simulink library "qrd_matrix_library"  (Simulink 8.7)
settings: Solver=ode45  StartTime=0.0  StopTime=10.0  RelTol=1e-3
values from neighbouring files (symbols this model uses):
  vectorization = 2    [qrd_test.m]
undefined symbols (not defined in the file or in its folder): AdvDSPBChannelOutDisplay, AdvDSPBDMemDisplay, Back_Substitution_instances, column_count, column_count_1, column_count_2, dpoly, dspba_ChannelInVis, dspba_ChannelOutVis, dspba_internal_get_channel_ports, evalAionMaskParam, latency, primtype, QRD_vectorization, recipsqrt, row, row_count, row_count_1, row_count_2, UseDontCare, value, x
libraries: DSPBAPrim x683, DSPBAControl x37, qrd_matrix_library x33, DSPBAVectorUtil x6, DSPBAVectorPrim x3
(part 4 of 8)

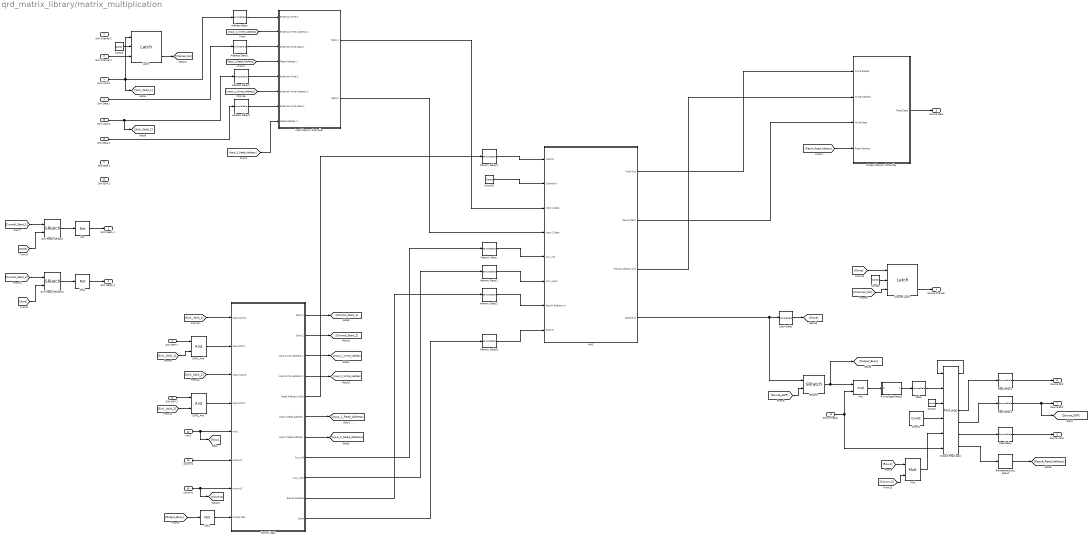
== system qrd_matrix_library/matrix_multiplication ==
  Sink Valid 1 : Inport
  Sink Channel 1 : Inport  Port=2
  Sink Data 1 : Inport  Port=3
  Sink SOP 1 : Inport  Port=4
  Sink EOP 1 : Inport  Port=5
  Sink Valid 2 : Inport  Port=6
  Sink Channel 2 : Inport  Port=7
  Sink Data 2 : Inport  Port=8
  Sink SOP 2 : Inport  Port=9
  Sink EOP 2 : Inport  Port=10
  Source Ready : Inport  Port=11
  row1 : Inport  Port=12
  column1 : Inport  Port=13
  column2 : Inport  Port=14
  Address Delay{,1..3} (4 alike) : DSPBAPrim/SampleDelay  primtype=sampdelay  nInputs=1  nOutputs=1  omode=Inherit via internal rule  otype=sfix(16)  scale=2^-15  rndmethod=Unbiased  factor=1  satmethod=Symmetric  shift_vec=[0 1 2 -1]  value=1  inPortNames=[' '; ' ';]  outPortNames=[' ']  dspbaimage=dspba_prim.jpg  text=dpoly(1, eye(1,value+1), 'z')  style=Optimised  visibilities=8 + 1024 + 2^17 + 2^18  flexible=off  slackgroup=0  augmented=0  version=20090407  advOptions=[]
  And : DSPBAPrim/And  primtype=and  nInputs=2  nOutputs=1  omode=Inherit via internal rule  otype=sfix(16)  scale=2^-15  rndmethod=Unbiased  factor=1  satmethod=Symmetric  shift_vec=[0 1 2 -1]  value=0  inPortNames=[' '; ' '; ' '; ' '; ' '; ' '; ' '; ' '; ' '; ' '; ' '; ' '; ' '; ' '; ' '; ' '; ]  outPortNames=[' ']  dspbaimage=dspba_prim.jpg  text=fprintf('&');  style=Optimised  visibilities=8+2  version=20090407
  Channel Latch : qrd_matrix_library/Latch
  Const1 : DSPBAPrim/Const  primtype=const  nInputs=0  nOutputs=1  omode=Inherit via internal rule  otype=uint(nextpow2(row*row))  scale=1  rndmethod=Unbiased  factor=1  satmethod=Symmetric  shift_vec=[0 1 2 -1]  value=1  inPortNames=['+'; '+';]  outPortNames=[' ']  dspbaimage=dspba_prim.jpg  text=fprintf('%s', num2str(value));  style=Optimised  visibilities=8 + 1024  floatPrecision=float32_m23  version=20120820
  Const2 : DSPBAPrim/Const  primtype=const  nInputs=0  nOutputs=1  omode=Specify via dialog  otype=uint(nextpow2(row_count_1*column_count_2))  scale=1  rndmethod=Unbiased  factor=1  satmethod=Symmetric  shift_vec=[0 1 2 -1]  value=0  inPortNames=['+'; '+';]  outPortNames=[' ']  dspbaimage=dspba_prim.jpg  text=fprintf('%s', num2str(value));  style=Optimised  visibilities=8 + 1024  floatPrecision=float32_m23  version=20120820
  Const26 : DSPBAPrim/Const  primtype=const  nInputs=0  nOutputs=1  omode=Specify via dialog  otype=uint(8)  scale=1  rndmethod=Unbiased  factor=1  satmethod=Symmetric  shift_vec=[0 1 2 -1]  value=0  inPortNames=['+'; '+';]  outPortNames=[' ']  dspbaimage=dspba_prim.jpg  text=fprintf('%s', num2str(value));  style=Optimised  visibilities=8 + 1024  floatPrecision=float32_m23  version=20120820
  Const6 : DSPBAPrim/Const  primtype=const  nInputs=0  nOutputs=1  omode=Specify via dialog  otype=uint(8)  scale=1  rndmethod=Unbiased  factor=1  satmethod=Symmetric  shift_vec=[0 1 2 -1]  value=0  inPortNames=['+'; '+';]  outPortNames=[' ']  dspbaimage=dspba_prim.jpg  text=fprintf('%s', num2str(value));  style=Optimised  visibilities=8 + 1024  floatPrecision=float32_m23  version=20120820
  Const8 : DSPBAPrim/Const  primtype=const  nInputs=0  nOutputs=1  omode=Specify via dialog  otype=uint(8)  scale=1  rndmethod=Unbiased  factor=1  satmethod=Symmetric  shift_vec=[0 1 2 -1]  value=0  inPortNames=['+'; '+';]  outPortNames=[' ']  dspbaimage=dspba_prim.jpg  text=fprintf('%s', num2str(value));  style=Optimised  visibilities=8 + 1024  floatPrecision=float32_m23  version=20120820
  Control Logic : Subsystem  BlockChoice=Row Major Control Logic
      settings: AttributesFormatString=%<BlockChoice>  TemplateBlock=qrd_matrix_library/Control Logic  MemberBlocks=Column Major Control Logic,Row Major Control Logic
  Delay : DSPBAPrim/SampleDelay  primtype=sampdelay  nInputs=1  nOutputs=1  omode=Inherit via internal rule  otype=sfix(16)  scale=2^-15  rndmethod=Unbiased  factor=1  satmethod=Symmetric  shift_vec=[0 1 2 -1]  value=1  inPortNames=[' '; ' ';]  outPortNames=[' ']  dspbaimage=dspba_prim.jpg  text=dpoly(1, eye(1,value+1), 'z')  style=Optimised  visibilities=8 + 1024 + 2^17 + 2^18  flexible=off  slackgroup=0  augmented=0  version=20090407  advOptions=[]
  Input Memory Controller : Subsystem
  Latch : qrd_matrix_library/Latch
  Latch Delay : DSPBAPrim/SampleDelay  primtype=sampdelay  nInputs=1  nOutputs=1  omode=Inherit via internal rule  otype=sfix(16)  scale=2^-15  rndmethod=Unbiased  factor=1  satmethod=Symmetric  shift_vec=[0 1 2 -1]  value=1  inPortNames=[' '; ' ';]  outPortNames=[' ']  dspbaimage=dspba_prim.jpg  text=dpoly(1, eye(1,value+1), 'z')  style=Optimised  visibilities=8 + 1024 + 2^17 + 2^18  flexible=off  slackgroup=0  augmented=0  version=20090407  advOptions=[]
  MAC : Subsystem
  Memory Delay{,1..2,4,6} (5 alike) : DSPBAPrim/SampleDelay  primtype=sampdelay  nInputs=1  nOutputs=1  omode=Inherit via internal rule  otype=sfix(16)  scale=2^-15  rndmethod=Unbiased  factor=1  satmethod=Symmetric  shift_vec=[0 1 2 -1]  value=2  inPortNames=[' '; ' ';]  outPortNames=[' ']  dspbaimage=dspba_prim.jpg  text=dpoly(1, eye(1,value+1), 'z')  style=Optimised  visibilities=8 + 1024 + 2^17 + 2^18  flexible=off  slackgroup=0  augmented=0  version=20090407  advOptions=[]
  Mult : DSPBAPrim/Mult  primtype=mult  nInputs=2  nOutputs=1  omode=Inherit via internal rule  otype=sfix(16)  scale=2^-15  rndmethod=Unbiased  factor=1  satmethod=Symmetric  shift_vec=[0 1 2 -1]  value=0  inPortNames=[' '; ' ';]  outPortNames=[' ']  dspbaimage=dspba_prim.jpg  text=fprintf('X');  style=Optimised  visibilities=8+2^18+2^19  floatPrecision=float32_m23  floatRounding=correct  advOptions=[]  version=20130115
  Not : DSPBAPrim/Not  primtype=not  nInputs=1  nOutputs=1  omode=Inherit via internal rule  otype=sfix(16)  scale=2^-15  rndmethod=Unbiased  factor=1  satmethod=Symmetric  shift_vec=[0 1 2 -1]  value=0  inPortNames=[' '; ' ';]  outPortNames=[' ']  dspbaimage=dspba_prim.jpg  text=fprintf('~');  style=Optimised  visibilities=8  version=20090407
  Not1 : DSPBAPrim/Not  primtype=not  nInputs=1  nOutputs=1  omode=Inherit via internal rule  otype=sfix(16)  scale=2^-15  rndmethod=Unbiased  factor=1  satmethod=Symmetric  shift_vec=[0 1 2 -1]  value=0  inPortNames=[' '; ' ';]  outPortNames=[' ']  dspbaimage=dspba_prim.jpg  text=fprintf('~');  style=Optimised  visibilities=8  version=20090407
  Not2 : DSPBAPrim/Not  primtype=not  nInputs=1  nOutputs=1  omode=Inherit via internal rule  otype=sfix(16)  scale=2^-15  rndmethod=Unbiased  factor=1  satmethod=Symmetric  shift_vec=[0 1 2 -1]  value=0  inPortNames=[' '; ' ';]  outPortNames=[' ']  dspbaimage=dspba_prim.jpg  text=fprintf('~');  style=Optimised  visibilities=8  version=20090407
  Output Memory Controller : Subsystem
  Output Read Logic : DSPBAPrim/ForLoop  looptest=<
  Read Delay : DSPBAPrim/SampleDelay  primtype=sampdelay  nInputs=1  nOutputs=1  omode=Inherit via internal rule  otype=sfix(16)  scale=2^-15  rndmethod=Unbiased  factor=1  satmethod=Symmetric  shift_vec=[0 1 2 -1]  value=2  inPortNames=[' '; ' ';]  outPortNames=[' ']  dspbaimage=dspba_prim.jpg  text=dpoly(1, eye(1,value+1), 'z')  style=Optimised  visibilities=8 + 1024 + 2^17 + 2^18  flexible=off  slackgroup=0  augmented=0  version=20090407  advOptions=[]
  Read Delay1 : DSPBAPrim/SampleDelay  primtype=sampdelay  nInputs=1  nOutputs=1  omode=Inherit via internal rule  otype=sfix(16)  scale=2^-15  rndmethod=Unbiased  factor=1  satmethod=Symmetric  shift_vec=[0 1 2 -1]  value=2  inPortNames=[' '; ' ';]  outPortNames=[' ']  dspbaimage=dspba_prim.jpg  text=dpoly(1, eye(1,value+1), 'z')  style=Optimised  visibilities=8 + 1024 + 2^17 + 2^18  flexible=off  slackgroup=0  augmented=0  version=20090407  advOptions=[]
  Read Delay2 : DSPBAPrim/SampleDelay  primtype=sampdelay  nInputs=1  nOutputs=1  omode=Inherit via internal rule  otype=sfix(16)  scale=2^-15  rndmethod=Unbiased  factor=1  satmethod=Symmetric  shift_vec=[0 1 2 -1]  value=2  inPortNames=[' '; ' ';]  outPortNames=[' ']  dspbaimage=dspba_prim.jpg  text=dpoly(1, eye(1,value+1), 'z')  style=Optimised  visibilities=8 + 1024 + 2^17 + 2^18  flexible=off  slackgroup=0  augmented=0  version=20090407  advOptions=[]
  ReinterpretCast_Result : DSPBAPrim/ReinterpretCast  primtype=reinterpret  nInputs=1  nOutputs=1  omode=Specify via dialog  otype=uint(nextpow2(row_count_1*column_count_2))  scale=1  rndmethod=Unbiased  factor=1  satmethod=Symmetric  shift_vec=[0 1 2 -1]  value=0  inPortNames=[' '; ' ';]  outPortNames=[' ']  dspbaimage=dspba_prim.jpg  text=fprintf('Reinterp\nCast', value);  style=Optimised  visibilities=8  floatPrecision=float32_m23  version=20120601
  Rising Edge Detect : Subsystem  Opaque=on
      mask help:
      | The EdgeDetect component detects edges,
      | under the assumption that initial state
      | of the signal is 0 i.e. a 1 on the input
      | in the first cycle will be detected as
      | an edge.
      mask Help: helpview(dspba.GetHelp('EdgeDetect'));
      mask Display:
      | color('w');
      | image(imread('dspba_fft.jpg'));
      | port_label('input',1,'d');
      | port_label('output',1,'q');
      | text(0.4,0.5,sprintf('RED'));
  SOP1_And : DSPBAPrim/And  primtype=and  nInputs=2  nOutputs=1  omode=Inherit via internal rule  otype=sfix(16)  scale=2^-15  rndmethod=Unbiased  factor=1  satmethod=Symmetric  shift_vec=[0 1 2 -1]  value=0  inPortNames=[' '; ' '; ' '; ' '; ' '; ' '; ' '; ' '; ' '; ' '; ' '; ' '; ' '; ' '; ' '; ' '; ]  outPortNames=[' ']  dspbaimage=dspba_prim.jpg  text=fprintf('&');  style=Optimised  visibilities=8+2  version=20090407
  SOP2_And : DSPBAPrim/And  primtype=and  nInputs=2  nOutputs=1  omode=Inherit via internal rule  otype=sfix(16)  scale=2^-15  rndmethod=Unbiased  factor=1  satmethod=Symmetric  shift_vec=[0 1 2 -1]  value=0  inPortNames=[' '; ' '; ' '; ' '; ' '; ' '; ' '; ' '; ' '; ' '; ' '; ' '; ' '; ' '; ' '; ' '; ]  outPortNames=[' ']  dspbaimage=dspba_prim.jpg  text=fprintf('&');  style=Optimised  visibilities=8+2  version=20090407
  SRlatch : DSPBAControl/SRlatch
  Sink Ready SRlatch : DSPBAControl/SRlatch
  Sink Ready SRlatch1 : DSPBAControl/SRlatch
  Sink Ready 1 : Outport
  Sink Ready 2 : Outport  Port=2
  Source Valid : Outport  Port=3
  Source Channel : Outport  Port=4
  Source Data : Outport  Port=5
  Source SOP : Outport  Port=6
  Source EOP : Outport  Port=7
  wires:
  Read Delay1/1 -> Source SOP/1
  Read Delay/1 -> Source Valid/1
  Control Logic/8(Acc_Init) -> Memory Delay/1
  Memory Delay2/1 -> MAC/7(Result Address In)
  Output Memory Controller/1(Read Data) -> Source Data/1
  Address Delay/1 -> Input Memory Controller/1(External Write 1)
  Sink Data 1/1 -> Address Delay1/1
  Memory Delay/1 -> MAC/5(Acc_Init)
  MAC/3(Result Address Out) -> Output Memory Controller/2(Write Address)
  Control Logic/10(Result Address) -> Memory Delay2/1
  MAC/2(Result Data) -> Output Memory Controller/3(Write Data)
  Control Logic/5(Read Address Valid) -> Memory Delay4/1
  Control Logic/3(Input Write Address 1) -> [Input_1_Write_Address]
  Address Delay1/1 -> Input Memory Controller/3(External Write Data 1)
  Source Ready/1 -> Output Read Logic/6, And/2
  [Input_1_Write_Address] -> Input Memory Controller/2(External Write Address 1)
  Memory Delay4/1 -> MAC/1(Valid In)
  Read Delay2/1 -> [Source_EOP], Source EOP/1
  Control Logic/9(Acc_Valid) -> Memory Delay1/1
  MAC/1(Valid Out) -> Output Memory Controller/1(Write Enable)
  [Result_Read_Address] -> Output Memory Controller/4(Read Address)
  Rising Edge Detect/1(q) -> Delay/1
  SRlatch/1 -> [Output_Busy], And/1
  Sink SOP 1/1 -> SOP1_And/1
  Const26/1 -> MAC/2(Channel In)
  Control Logic/6(Input 1 Read Address) -> [Input_1_Read_Address]
  [Input_1_Read_Address] -> Input Memory Controller/4(Read Address 1)
  [Input_2_Read_Address] -> Input Memory Controller/8(Read Address 2)
  And/1 -> Rising Edge Detect/1(d)
  Memory Delay1/1 -> MAC/6(Acc_Valid)
  Input Memory Controller/2(Data 2) -> MAC/4(Input 2 Data)
  Input Memory Controller/1(Data 1) -> MAC/3(Input 1 Data)
  Sink Valid 1/1 -> [Sink_Valid_1], Address Delay/1, Latch/1
  Delay/1 -> Output Read Logic/2
  MAC/4(Done Out) -> Latch Delay/1, SRlatch/1
  Output Read Logic/6 -> Read Delay/1
  Output Read Logic/7 -> ReinterpretCast_Result/1
  Output Read Logic/4 -> Read Delay1/1
  Output Read Logic/5 -> Read Delay2/1
  Mult/1 -> Output Read Logic/5
  Const1/1 -> Output Read Logic/4
  Const2/1 -> Output Read Logic/3
  Output Read Logic/1 -> Output Read Logic/1
  Control Logic/11(Done) -> Memory Delay6/1
  Memory Delay6/1 -> MAC/8(Done In)
  [Source_EOP] -> SRlatch/2
  row1/1 -> [Row1], Control Logic/5(row1)
  column1/1 -> Control Logic/6(column1)
  Not/1 -> Sink Ready 1/1
  [Done] -> Sink Ready SRlatch/2
  [Row1] -> Mult/1
  Sink Channel 1/1 -> Latch/3
  Const6/1 -> Latch/2
  Latch/3 -> [Channel_Out]
  Sink Ready SRlatch/1 -> Not/1
  [Sink_Valid_1] -> SOP1_And/2
  SOP1_And/1 -> Control Logic/2(Input SOP 1)
  Control Logic/1(Start 1) -> [Control_Start_1]
  [Control_Start_1] -> Sink Ready SRlatch/1
  Not1/1 -> Sink Ready 2/1
  [Done] -> Sink Ready SRlatch1/2
  Sink Ready SRlatch1/1 -> Not1/1
  [Control_Start_2] -> Sink Ready SRlatch1/1
  Address Delay2/1 -> Input Memory Controller/5(External Write 2)
  Sink Valid 2/1 -> [Sink_Valid_2], Address Delay2/1
  Address Delay3/1 -> Input Memory Controller/7(External Write Data 2)
  Sink Data 2/1 -> Address Delay3/1
  [Sink_Valid_2] -> SOP2_And/2
  Sink SOP 2/1 -> SOP2_And/1
  [Sink_Valid_1] -> Control Logic/1(Input Valid 1)
  [Sink_Valid_2] -> Control Logic/3(Input Valid 2)
  SOP2_And/1 -> Control Logic/4(Input SOP 2)
  column2/1 -> [Column2], Control Logic/7(column2)
  [Column2] -> Mult/2
  Control Logic/2(Start 2) -> [Control_Start_2]
  [Input_2_Write_Address] -> Input Memory Controller/6(External Write Address 2)
  Control Logic/4(Input Write Address 2) -> [Input_2_Write_Address]
  Control Logic/7(Input 2 Read Address) -> [Input_2_Read_Address]
  ReinterpretCast_Result/1 -> [Result_Read_Address]
  [Output_Busy] -> Not2/1
  Latch Delay/1 -> [Done]
  Not2/1 -> Control Logic/8(Output Idle)
  [Channel_Out] -> Channel Latch/3
  Const8/1 -> Channel Latch/2
  [Done] -> Channel Latch/1
  Channel Latch/3 -> Source Channel/1

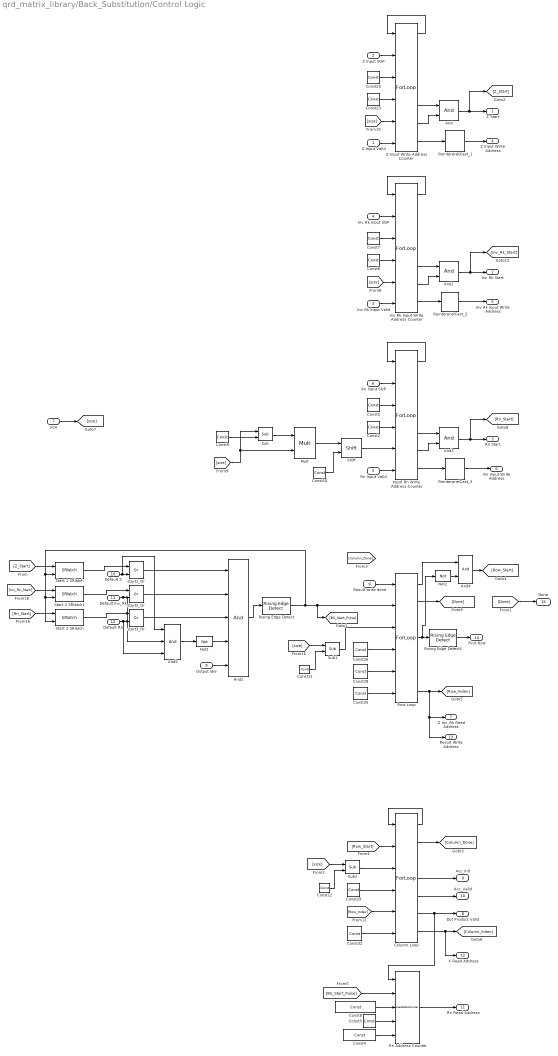
== system qrd_matrix_library/Back_Substitution/Control Logic ==
  Z Input Valid : Inport
  Z Input SOP : Inport  Port=2
  Inv Rk Input Valid : Inport  Port=3
  Inv Rk Input SOP : Inport  Port=4
  Rn Input Valid : Inport  Port=5
  Rn Input SOP : Inport  Port=6
  size : Inport  Port=7
  Output Idle : Inport  Port=8
  Result write done : Inport  Port=9
  Default Z : Inport  Port=10
  Default Inv_Rk : Inport  Port=11
  Default Rn : Inport  Port=12
  And{,1,3..4} (4 alike) : DSPBAPrim/And  primtype=and  nInputs=2  nOutputs=1  omode=Inherit via internal rule  otype=sfix(16)  scale=2^-15  rndmethod=Unbiased  factor=1  satmethod=Symmetric  shift_vec=[0 1 2 -1]  value=0  inPortNames=[' '; ' '; ' '; ' '; ' '; ' '; ' '; ' '; ' '; ' '; ' '; ' '; ' '; ' '; ' '; ' '; ]  outPortNames=[' ']  dspbaimage=dspba_prim.jpg  text=fprintf('&');  style=Optimised  visibilities=8+2  version=20090407
  And2 : DSPBAPrim/And  primtype=and  nInputs=5  nOutputs=1  omode=Inherit via internal rule  otype=sfix(16)  scale=2^-15  rndmethod=Unbiased  factor=1  satmethod=Symmetric  shift_vec=[0 1 2 -1]  value=0  inPortNames=[' '; ' '; ' '; ' '; ' '; ' '; ' '; ' '; ' '; ' '; ' '; ' '; ' '; ' '; ' '; ' '; ]  outPortNames=[' ']  dspbaimage=dspba_prim.jpg  text=fprintf('&');  style=Optimised  visibilities=8+2  version=20090407
  And5 : DSPBAPrim/And  primtype=and  nInputs=3  nOutputs=1  omode=Inherit via internal rule  otype=sfix(16)  scale=2^-15  rndmethod=Unbiased  factor=1  satmethod=Symmetric  shift_vec=[0 1 2 -1]  value=0  inPortNames=[' '; ' '; ' '; ' '; ' '; ' '; ' '; ' '; ' '; ' '; ' '; ' '; ' '; ' '; ' '; ' '; ]  outPortNames=[' ']  dspbaimage=dspba_prim.jpg  text=fprintf('&');  style=Optimised  visibilities=8+2  version=20090407
  Column Loop : DSPBAPrim/ForLoop  looptest=>
  Const10 : DSPBAPrim/Const  primtype=const  nInputs=0  nOutputs=1  omode=Inherit via internal rule  otype=uint(nextpow2(row*row))  scale=1  rndmethod=Unbiased  factor=1  satmethod=Symmetric  shift_vec=[0 1 2 -1]  value=1  inPortNames=['+'; '+';]  outPortNames=[' ']  dspbaimage=dspba_prim.jpg  text=fprintf('%s', num2str(value));  style=Optimised  visibilities=8 + 1024  floatPrecision=float32_m23  version=20120820
  Const{2,6,11..12,23,35} (6 alike) : DSPBAPrim/Const  primtype=const  nInputs=0  nOutputs=1  omode=Inherit via internal rule  otype=uint(8)  scale=1  rndmethod=Unbiased  factor=1  satmethod=Symmetric  shift_vec=[0 1 2 -1]  value=1  inPortNames=['+'; '+';]  outPortNames=[' ']  dspbaimage=dspba_prim.jpg  text=fprintf('%s', num2str(value));  style=Optimised  visibilities=8 + 1024  floatPrecision=float32_m23  version=20120820
  Const{5,7,25,28} (4 alike) : DSPBAPrim/Const  primtype=const  nInputs=0  nOutputs=1  omode=Inherit via internal rule  otype=uint(8)  scale=1  rndmethod=Unbiased  factor=1  satmethod=Symmetric  shift_vec=[0 1 2 -1]  value=0  inPortNames=['+'; '+';]  outPortNames=[' ']  dspbaimage=dspba_prim.jpg  text=fprintf('%s', num2str(value));  style=Optimised  visibilities=8 + 1024  floatPrecision=float32_m23  version=20120820
  Const26 : DSPBAPrim/Const  primtype=const  nInputs=0  nOutputs=1  omode=Inherit via internal rule  otype=uint(8)  scale=1  rndmethod=Unbiased  factor=1  satmethod=Symmetric  shift_vec=[0 1 2 -1]  value=-1  inPortNames=['+'; '+';]  outPortNames=[' ']  dspbaimage=dspba_prim.jpg  text=fprintf('%s', num2str(value));  style=Optimised  visibilities=8 + 1024  floatPrecision=float32_m23  version=20120820
  Const29 : DSPBAPrim/Const  primtype=const  nInputs=0  nOutputs=1  omode=Inherit via internal rule  otype=uint(8)  scale=1  rndmethod=Unbiased  factor=1  satmethod=Symmetric  shift_vec=[0 1 2 -1]  value=-1  inPortNames=['+'; '+';]  outPortNames=[' ']  dspbaimage=dspba_prim.jpg  text=fprintf('%s', num2str(value));  style=Optimised  visibilities=8 + 1024  floatPrecision=float32_m23  version=20120820
  Const3 : DSPBAPrim/Const  primtype=const  nInputs=0  nOutputs=1  omode=Inherit via internal rule  otype=uint(8)  scale=1  rndmethod=Unbiased  factor=1  satmethod=Symmetric  shift_vec=[0 1 2 -1]  value=-1  inPortNames=['+'; '+';]  outPortNames=[' ']  dspbaimage=dspba_prim.jpg  text=fprintf('%s', num2str(value));  style=Optimised  visibilities=8 + 1024  floatPrecision=float32_m23  version=20120820
  Const32 : DSPBAPrim/Const  primtype=const  nInputs=0  nOutputs=1  omode=boolean  otype=uint(8)  scale=1  rndmethod=Unbiased  factor=1  satmethod=Symmetric  shift_vec=[0 1 2 -1]  value=1  inPortNames=['+'; '+';]  outPortNames=[' ']  dspbaimage=dspba_prim.jpg  text=fprintf('%s', num2str(value));  style=Optimised  visibilities=8 + 1024  floatPrecision=float32_m23  version=20120820
  Const4 : DSPBAPrim/Const  primtype=const  nInputs=0  nOutputs=1  omode=Inherit via internal rule  otype=uint(8)  scale=1  rndmethod=Unbiased  factor=1  satmethod=Symmetric  shift_vec=[0 1 2 -1]  value=(size-1)*size/2  inPortNames=['+'; '+';]  outPortNames=[' ']  dspbaimage=dspba_prim.jpg  text=fprintf('%s', num2str(value));  style=Optimised  visibilities=8 + 1024  floatPrecision=float32_m23  version=20120820
  Const8 : DSPBAPrim/Const  primtype=const  nInputs=0  nOutputs=1  omode=Inherit via internal rule  otype=uint(8)  scale=1  rndmethod=Unbiased  factor=1  satmethod=Symmetric  shift_vec=[0 1 2 -1]  value=((size-1)*size/2)-1  inPortNames=['+'; '+';]  outPortNames=[' ']  dspbaimage=dspba_prim.jpg  text=fprintf('%s', num2str(value));  style=Optimised  visibilities=8 + 1024  floatPrecision=float32_m23  version=20120820
  Const9 : DSPBAPrim/Const  primtype=const  nInputs=0  nOutputs=1  omode=Inherit via internal rule  otype=uint(nextpow2(row*row))  scale=1  rndmethod=Unbiased  factor=1  satmethod=Symmetric  shift_vec=[0 1 2 -1]  value=1  inPortNames=['+'; '+';]  outPortNames=[' ']  dspbaimage=dspba_prim.jpg  text=fprintf('%s', num2str(value));  style=Optimised  visibilities=8 + 1024  floatPrecision=float32_m23  version=20120820
  Input Rn Write Address Counter : DSPBAPrim/ForLoop  looptest=<
  Inv Rk Input Write Address Counter : DSPBAPrim/ForLoop  looptest=<
  Mult : DSPBAPrim/Mult  primtype=mult  nInputs=2  nOutputs=1  omode=Inherit via internal rule  otype=sfix(16)  scale=2^-15  rndmethod=Unbiased  factor=1  satmethod=Symmetric  shift_vec=[0 1 2 -1]  value=0  inPortNames=[' '; ' ';]  outPortNames=[' ']  dspbaimage=dspba_prim.jpg  text=fprintf('X');  style=Optimised  visibilities=8+2^18+2^19  floatPrecision=float32_m23  floatRounding=correct  advOptions=[]  version=20130115
  Not1 : DSPBAPrim/Not  primtype=not  nInputs=1  nOutputs=1  omode=Inherit via internal rule  otype=sfix(16)  scale=2^-15  rndmethod=Unbiased  factor=1  satmethod=Symmetric  shift_vec=[0 1 2 -1]  value=0  inPortNames=[' '; ' ';]  outPortNames=[' ']  dspbaimage=dspba_prim.jpg  text=fprintf('~');  style=Optimised  visibilities=8  version=20090407
  Not2 : DSPBAPrim/Not  primtype=not  nInputs=1  nOutputs=1  omode=Inherit via internal rule  otype=sfix(16)  scale=2^-15  rndmethod=Unbiased  factor=1  satmethod=Symmetric  shift_vec=[0 1 2 -1]  value=0  inPortNames=[' '; ' ';]  outPortNames=[' ']  dspbaimage=dspba_prim.jpg  text=fprintf('~');  style=Optimised  visibilities=8  version=20090407
  ReinterpretCast_1 : DSPBAPrim/ReinterpretCast  primtype=reinterpret  nInputs=1  nOutputs=1  omode=Specify via dialog  otype=uint(nextpow2(size))  scale=1  rndmethod=Unbiased  factor=1  satmethod=Symmetric  shift_vec=[0 1 2 -1]  value=0  inPortNames=[' '; ' ';]  outPortNames=[' ']  dspbaimage=dspba_prim.jpg  text=fprintf('Reinterp\nCast', value);  style=Optimised  visibilities=8  floatPrecision=float32_m23  version=20120601
  ReinterpretCast_2 : DSPBAPrim/ReinterpretCast  primtype=reinterpret  nInputs=1  nOutputs=1  omode=Specify via dialog  otype=uint(nextpow2(size))  scale=1  rndmethod=Unbiased  factor=1  satmethod=Symmetric  shift_vec=[0 1 2 -1]  value=0  inPortNames=[' '; ' ';]  outPortNames=[' ']  dspbaimage=dspba_prim.jpg  text=fprintf('Reinterp\nCast', value);  style=Optimised  visibilities=8  floatPrecision=float32_m23  version=20120601
  ReinterpretCast_3 : DSPBAPrim/ReinterpretCast  primtype=reinterpret  nInputs=1  nOutputs=1  omode=Specify via dialog  otype=uint(nextpow2(((size-1)*size/2)))  scale=1  rndmethod=Unbiased  factor=1  satmethod=Symmetric  shift_vec=[0 1 2 -1]  value=0  inPortNames=[' '; ' ';]  outPortNames=[' ']  dspbaimage=dspba_prim.jpg  text=fprintf('Reinterp\nCast', value);  style=Optimised  visibilities=8  floatPrecision=float32_m23  version=20120601
  Rising Edge Detect : qrd_matrix_library/matrix_multiplication/Rising Edge Detect
  Rising Edge Detect1 : qrd_matrix_library/matrix_multiplication/Rising Edge Detect
  Rn Address Counter : DSPBAPrim/LoadableCounter  primtype=loadablecounter  nInputs=5  nOutputs=1  omode=Inherit via internal rule  otype=ufix(16)  scale=2^-0  rndmethod=Unbiased  factor=1  satmethod=Symmetric  shift_vec=[0 1 2 -1]  value=[((size-1)*size/2)-1 ((size-1)*size/2) -1]  inPortNames=['en';'ld';'i ';'s ';'m ']  outPortNames=[' ']  dspbaimage=dspba_prim.jpg  text=fprintf('loadable\ncounter\n[%d %d %d]', value(1), value(2), value(3));  style=Optimised  visibilities=8 + 1024  version=20090407
  Row Loop : DSPBAPrim/ForLoop  looptest=>=
  Shift : DSPBAPrim/Shift  primtype=shift  nInputs=2  nOutputs=1  omode=Inherit via internal rule  otype=uint(nextpow2(((size-1)*size/2)))  scale=1  rndmethod=Unbiased  factor=1  satmethod=Symmetric  shift_vec=[0 1 2 -1]  value=0  inPortNames=['a'; 'b';]  outPortNames=[' ']  dspbaimage=dspba_prim.jpg  text=fprintf('a >> b');  style=Optimised  visibilities=8  version=20090407
  Start 1 SRlatch : DSPBAControl/SRlatch
  Start 2 SRlatch1 : DSPBAControl/SRlatch
  Start 3 SRlatch : DSPBAControl/SRlatch
  Sub : DSPBAPrim/Sub  primtype=sub  nInputs=2  nOutputs=1  omode=Specify via dialog  otype=uint(nextpow2(size))  scale=1  rndmethod=Unbiased  factor=1  satmethod=Symmetric  shift_vec=[0 1 2 -1]  value=0  inPortNames=['+'; '-';]  outPortNames=[' ']  dspbaimage=dspba_prim.jpg  text=fprintf('-');  style=Optimised  visibilities=8+2^17+2^18  floatRounding=correct  advOptions=[]  version=20130115
  Sub1 : DSPBAPrim/Sub  primtype=sub  nInputs=2  nOutputs=1  omode=Inherit via internal rule with word growth  otype=sfix(16)  scale=2^-15  rndmethod=Unbiased  factor=1  satmethod=Symmetric  shift_vec=[0 1 2 -1]  value=0  inPortNames=['+'; '-';]  outPortNames=[' ']  dspbaimage=dspba_prim.jpg  text=fprintf('-');  style=Optimised  visibilities=8+2^17+2^18  floatRounding=correct  advOptions=[]  version=20130115
  Sub2 : DSPBAPrim/Sub  primtype=sub  nInputs=2  nOutputs=1  omode=Inherit via internal rule with word growth  otype=sfix(16)  scale=2^-15  rndmethod=Unbiased  factor=1  satmethod=Symmetric  shift_vec=[0 1 2 -1]  value=0  inPortNames=['+'; '-';]  outPortNames=[' ']  dspbaimage=dspba_prim.jpg  text=fprintf('-');  style=Optimised  visibilities=8+2^17+2^18  floatRounding=correct  advOptions=[]  version=20130115
  Z Input Write Address Counter : DSPBAPrim/ForLoop  looptest=<
  start1_Or : DSPBAPrim/Or  primtype=or  nInputs=2  nOutputs=1  omode=Inherit via internal rule  otype=sfix(16)  scale=2^-15  rndmethod=Unbiased  factor=1  satmethod=Symmetric  shift_vec=[0 1 2 -1]  value=0  inPortNames=[' '; ' '; ' '; ' '; ' '; ' '; ' '; ' '; ' '; ' '; ' '; ' '; ' '; ' '; ' '; ' '; ]  outPortNames=[' ']  dspbaimage=dspba_prim.jpg  text=fprintf('|');  style=Optimised  visibilities=8+2  version=20090407
  start2_Or : DSPBAPrim/Or  primtype=or  nInputs=2  nOutputs=1  omode=Inherit via internal rule  otype=sfix(16)  scale=2^-15  rndmethod=Unbiased  factor=1  satmethod=Symmetric  shift_vec=[0 1 2 -1]  value=0  inPortNames=[' '; ' '; ' '; ' '; ' '; ' '; ' '; ' '; ' '; ' '; ' '; ' '; ' '; ' '; ' '; ' '; ]  outPortNames=[' ']  dspbaimage=dspba_prim.jpg  text=fprintf('|');  style=Optimised  visibilities=8+2  version=20090407
  start3_Or : DSPBAPrim/Or  primtype=or  nInputs=2  nOutputs=1  omode=Inherit via internal rule  otype=sfix(16)  scale=2^-15  rndmethod=Unbiased  factor=1  satmethod=Symmetric  shift_vec=[0 1 2 -1]  value=0  inPortNames=[' '; ' '; ' '; ' '; ' '; ' '; ' '; ' '; ' '; ' '; ' '; ' '; ' '; ' '; ' '; ' '; ]  outPortNames=[' ']  dspbaimage=dspba_prim.jpg  text=fprintf('|');  style=Optimised  visibilities=8+2  version=20090407
  Z Start : Outport
  Inv Rk Start : Outport  Port=2
  Rn Start : Outport  Port=3
  Z Input Write Address : Outport  Port=4
  Inv Rk Input Write Address : Outport  Port=5
  Rn Input Write Address : Outport  Port=6
  Z Inv_Rk Read Address : Outport  Port=7
  Dot Product Valid : Outport  Port=8
  Acc_Init : Outport  Port=9
  Acc_Valid : Outport  Port=10
  Rn Read Address : Outport  Port=11
  X Read Address : Outport  Port=12
  Result Write Address : Outport  Port=13
  First Row : Outport  Port=14
  Done : Outport  Port=15
  wires:
  Z Input SOP/1 -> Z Input Write Address Counter/2
  Z Input Write Address Counter/6 -> And/2
  Z Input Write Address Counter/5 -> And/1
  Z Input Write Address Counter/1 -> Z Input Write Address Counter/1
  Z Input Valid/1 -> Z Input Write Address Counter/6
  size/1 -> [size]
  Row Loop/2 -> [Done]
  Column Loop/7 -> X Read Address/1, [Column_Index]
  Row Loop/1 -> And4/1
  [Row_Start] -> Column Loop/2
  Result write done/1 -> Row Loop/1
  Column Loop/2 -> [Column_Done]
  Column Loop/1 -> Column Loop/1
  Const35/1 -> Row Loop/6
  Const32/1 -> Column Loop/6
  Row Loop/7 -> Result Write Address/1, Z Inv_Rk Read Address/1, [Row_Index]
  Rising Edge Detect/1 -> [BS_Start_Pulse], Row Loop/2, Start 1 SRlatch/2, Start 3 SRlatch/2, Start 2 SRlatch1/2
  Const29/1 -> Column Loop/4
  [Row_Index] -> Column Loop/5
  Const26/1 -> Row Loop/4
  Const28/1 -> Row Loop/5
  Z Input Write Address Counter/7 -> ReinterpretCast_1/1
  Const25/1 -> Z Input Write Address Counter/3
  Const23/1 -> Z Input Write Address Counter/4
  Inv Rk Input SOP/1 -> Inv Rk Input Write Address Counter/2
  Inv Rk Input Write Address Counter/6 -> And1/2
  Inv Rk Input Write Address Counter/5 -> And1/1
  Inv Rk Input Write Address Counter/1 -> Inv Rk Input Write Address Counter/1
  Inv Rk Input Valid/1 -> Inv Rk Input Write Address Counter/6
  Inv Rk Input Write Address Counter/7 -> ReinterpretCast_2/1
  Const7/1 -> Inv Rk Input Write Address Counter/3
  Const6/1 -> Inv Rk Input Write Address Counter/4
  And/1 -> [Z_Start], Z Start/1
  And1/1 -> [Inv_Rk_Start], Inv Rk Start/1
  [Z_Start] -> Start 1 SRlatch/1
  [Inv_Rk_Start] -> Start 2 SRlatch1/1
  And2/1 -> Rising Edge Detect/1
  Sub2/1 -> Column Loop/3
  ReinterpretCast_1/1 -> Z Input Write Address/1
  ReinterpretCast_2/1 -> Inv Rk Input Write Address/1
  Start 3 SRlatch/1 -> start3_Or/1
  Start 1 SRlatch/1 -> start1_Or/1
  Start 2 SRlatch1/1 -> start2_Or/1
  [size] -> Z Input Write Address Counter/5
  [size] -> Inv Rk Input Write Address Counter/5
  Rn Input SOP/1 -> Input Rn Write Address Counter/2
  Input Rn Write Address Counter/6 -> And3/2
  Input Rn Write Address Counter/5 -> And3/1
  Input Rn Write Address Counter/1 -> Input Rn Write Address Counter/1
  Rn Input Valid/1 -> Input Rn Write Address Counter/6
  Input Rn Write Address Counter/7 -> ReinterpretCast_3/1
  Const5/1 -> Input Rn Write Address Counter/3
  Const2/1 -> Input Rn Write Address Counter/4
  And3/1 -> Rn Start/1, [Rn_Start]
  ReinterpretCast_3/1 -> Rn Input Write Address/1
  Shift/1 -> Input Rn Write Address Counter/5
  Mult/1 -> Shift/1
  [size] -> Sub/1, Mult/2
  Sub/1 -> Mult/1
  Const9/1 -> Sub/2
  Const10/1 -> Shift/2
  Not1/1 -> And2/4
  [Rn_Start] -> Start 3 SRlatch/1
  [size] -> Sub1/1
  Sub1/1 -> Row Loop/3
  Const11/1 -> Sub1/2
  [size] -> Sub2/1
  Const12/1 -> Sub2/2
  [Done] -> Done/1
  Column Loop/6 -> Rn Address Counter/1, Dot Product Valid/1
  Const3/1 -> Rn Address Counter/4
  Const4/1 -> Rn Address Counter/5
  Const8/1 -> Rn Address Counter/3
  [BS_Start_Pulse] -> Rn Address Counter/2
  Rn Address Counter/1 -> Rn Read Address/1
  Row Loop/4 -> Not2/1, Rising Edge Detect1/1
  Rising Edge Detect1/1 -> First Row/1
  Not2/1 -> And4/2
  And4/1 -> [Row_Start]
  Column Loop/4 -> Acc_Init/1
  Column Loop/5 -> Acc_Valid/1
  Default Z/1 -> And5/1, start1_Or/2
  start1_Or/1 -> And2/1
  start2_Or/1 -> And2/2
  Default Inv_Rk/1 -> And5/2, start2_Or/2
  Default Rn/1 -> And5/3, start3_Or/2
  start3_Or/1 -> And2/3
  Output Idle/1 -> And2/5
  And5/1 -> Not1/1

== system qrd_matrix_library/Back_Substitution/Data Mux ==
  Valid In : Inport
  Channel In : Inport  Port=2
  Dot_Product_valid_in : Inport  Port=3
  Divide_valid_in : Inport  Port=4
  First_Column_in : Inport  Port=5
  Rn_Data : Inport  Port=6
  X_Data : Inport  Port=7
  Sub_Data : Inport  Port=8
  Inv_Rk_Data : Inport  Port=9
  Acc_Init_In : Inport  Port=10
  Acc_Valid_In : Inport  Port=11
  Z_Data_In : Inport  Port=12
  ChannelIn : DSPBAPrim/ChannelIn  primtype=channelin  nInputs=dspba_internal_get_channel_ports(gcb)  nOutputs=dspba_internal_get_channel_ports(gcb)  omode=Inherit via internal rule  otype=sfix(16)  scale=2^-15  rndmethod=Unbiased  factor=1  satmethod=Symmetric  shift_vec=[0 1 2 -1]  value=10  inPortNames=['v'; 'c'; '0'; '1'; '2'; '3'; '4'; '5'; '6'; '7'; '8'; '9'; 'A'; 'B'; 'D'; 'E'; 'F'; 'G'; 'H'; 'I'; 'J'; 'K'; 'L'; 'M'; 'N'; 'O'; 'P'; 'Q'; 'R'; 'S'; 'T'; 'U'; 'W'; 'X'; 'Y'; 'Z']  outPortNames=['v'; 'c'; '0'; '1'; '2'; '3'; '4'; '5'; '6'; '7'; '8'; '9'; 'A'; 'B'; 'D'; 'E'; 'F'; 'G'; 'H'; 'I'; 'J'; 'K'; 'L'; 'M'; 'N'; 'O'; 'P'; 'Q'; 'R'; 'S'; 'T'; 'U'; 'W'; 'X'; 'Y'; 'Z']  dspbaimage=dspba_prim.jpg  text=fprintf('In');  style=Optimised  dataSignals=10  foldingEnabled=off  channels=1  sampleRate=200  packetBeginPresent=off  packetBeginEnabled=off  visibilities=dspba_ChannelInVis(gcb)  latencyCorrection=0  version=20141013
  ChannelOut : DSPBAPrim/ChannelOut  primtype=channelout  nInputs=dspba_internal_get_channel_ports(gcb)  nOutputs=dspba_internal_get_channel_ports(gcb)  omode=Inherit via internal rule  otype=sfix(16)  scale=2^-15  rndmethod=Unbiased  factor=1  satmethod=Symmetric  shift_vec=[0 1 2 -1]  value=6  inPortNames=['v'; 'c'; '0'; '1'; '2'; '3'; '4'; '5'; '6'; '7'; '8'; '9'; 'A'; 'B'; 'D'; 'E'; 'F'; 'G'; 'H'; 'I'; 'J'; 'K'; 'L'; 'M'; 'N'; 'O'; 'P'; 'Q'; 'R'; 'S'; 'T'; 'U'; 'W'; 'X'; 'Y'; 'Z']  outPortNames=['v'; 'c'; '0'; '1'; '2'; '3'; '4'; '5'; '6'; '7'; '8'; '9'; 'A'; 'B'; 'D'; 'E'; 'F'; 'G'; 'H'; 'I'; 'J'; 'K'; 'L'; 'M'; 'N'; 'O'; 'P'; 'Q'; 'R'; 'S'; 'T'; 'U'; 'W'; 'X'; 'Y'; 'Z']  dspbaimage=dspba_prim.jpg  text=fprintf('Out%s', AdvDSPBChannelOutDisplay(latency));  style=Optimised  dataSignals=6  foldingEnabled=off  channels=1  sampleRate=200  packetBeginPresent=off  packetBeginEnabled=off  visibilities=dspba_ChannelOutVis(gcb)  latency=0  latencyCorrection=0  version=20141013
  Data1 Select : DSPBAPrim/Select  primtype=select  nInputs=str2num(get_param(gcb,'value'))*2+1  nOutputs=1  omode=Inherit via internal rule  otype=sfix(16)  scale=2^-15  rndmethod=Unbiased  factor=1  satmethod=Symmetric  shift_vec=[0 1 2 -1]  value=2  inPortNames=['d'; '0'; 'a'; '1'; 'b'; '2'; 'c'; '3'; 'd'; '4'; 'e'; '5'; 'f'; '6'; 'g'; '7'; 'h'; '8'; 'i'; '9'; 'j']  outPortNames=[' ']  dspbaimage=dspba_prim.jpg  text=fprintf('%s', primtype);  style=Optimised  visibilities=8 + 1024  version=20090407
  Data2 Select : DSPBAPrim/Select  primtype=select  nInputs=str2num(get_param(gcb,'value'))*2+1  nOutputs=1  omode=Inherit via internal rule  otype=sfix(16)  scale=2^-15  rndmethod=Unbiased  factor=1  satmethod=Symmetric  shift_vec=[0 1 2 -1]  value=2  inPortNames=['d'; '0'; 'a'; '1'; 'b'; '2'; 'c'; '3'; 'd'; '4'; 'e'; '5'; 'f'; '6'; 'g'; '7'; 'h'; '8'; 'i'; '9'; 'j']  outPortNames=[' ']  dspbaimage=dspba_prim.jpg  text=fprintf('%s', primtype);  style=Optimised  visibilities=8 + 1024  version=20090407
  SynthesisInfo : DSPBAPrim/SynthesisInfo  primtype=synthinfo  nInputs=0  nOutputs=0  omode=Inherit via internal rule  otype=sfix(16)  scale=2^-15  rndmethod=Truncate  factor=1  satmethod=Symmetric  shift_vec=[0 1 2 -1]  value=99  inPortNames=[' '; ' ';]  outPortNames=[' ']  dspbaimage=dspba_prim_ctrl.jpg  text=fprintf('Style=%s', style);  style=Scheduled  visibilities=2^17+2^18+2^19+2^20  constraintInUse=off  constraintRelation=>  constraintLimit=2  bitAccurate=off  version=20150220
  Valid_Or : DSPBAPrim/Or  primtype=or  nInputs=2  nOutputs=1  omode=Inherit via internal rule  otype=sfix(16)  scale=2^-15  rndmethod=Unbiased  factor=1  satmethod=Symmetric  shift_vec=[0 1 2 -1]  value=0  inPortNames=[' '; ' '; ' '; ' '; ' '; ' '; ' '; ' '; ' '; ' '; ' '; ' '; ' '; ' '; ' '; ' '; ]  outPortNames=[' ']  dspbaimage=dspba_prim.jpg  text=fprintf('|');  style=Optimised  visibilities=8+2  version=20090407
  Valid Out : Outport
  Data Out 1 : Outport  Port=2
  Data Out 2 : Outport  Port=3
  Acc_Init_Out : Outport  Port=4
  Acc_Valid_Out : Outport  Port=5
  Dot_Product_valid_out : Outport  Port=6
  Divide_Valid_Out : Outport  Port=7
  wires:
  First_Column_in/1 -> ChannelIn/5
  Divide_valid_in/1 -> ChannelIn/4
  Dot_Product_valid_in/1 -> ChannelIn/3
  Sub_Data/1 -> ChannelIn/8
  ChannelOut/1 -> Valid Out/1
  ChannelOut/4 -> Data Out 2/1
  Channel In/1 -> ChannelIn/2
  ChannelOut/5 -> Acc_Init_Out/1
  ChannelOut/3 -> Data Out 1/1
  Data1 Select/1 -> ChannelOut/3
  ChannelOut/6 -> Acc_Valid_Out/1
  Z_Data_In/1 -> ChannelIn/10
  Data2 Select/1 -> ChannelOut/4
  Inv_Rk_Data/1 -> ChannelIn/9
  X_Data/1 -> ChannelIn/7
  Rn_Data/1 -> ChannelIn/6
  Valid In/1 -> ChannelIn/1
  ChannelIn/1 -> ChannelOut/1
  ChannelIn/2 -> ChannelOut/2
  ChannelIn/3 -> Data1 Select/2, ChannelOut/7, Data2 Select/2
  ChannelIn/4 -> Data1 Select/4, Valid_Or/2, Data2 Select/4
  ChannelIn/6 -> Data1 Select/3
  ChannelIn/7 -> Data2 Select/3
  ChannelIn/8 -> Data1 Select/5
  ChannelIn/9 -> Data2 Select/1, Data2 Select/5
  ChannelIn/11 -> ChannelOut/5
  ChannelIn/12 -> ChannelOut/6
  ChannelOut/7 -> Dot_Product_valid_out/1
  Acc_Init_In/1 -> ChannelIn/11
  ChannelIn/5 -> Valid_Or/1
  Valid_Or/1 -> ChannelOut/8
  Acc_Valid_In/1 -> ChannelIn/12
  ChannelIn/10 -> Data1 Select/1
  ChannelOut/8 -> Divide_Valid_Out/1

== system qrd_matrix_library/Back_Substitution/Dot Product ==
  Valid_In : Inport
  Channel_In : Inport  Port=2
  Data_In1 : Inport  Port=3
  Data_In2 : Inport  Port=4
  Acc_Init : Inport  Port=5
  Acc_Valid : Inport  Port=6
  Dot_Product_Valid_In : Inport  Port=7
  Mult_Valid_In : Inport  Port=8
  Acc : DSPBAPrim/Acc  primtype=acc  nInputs=2  nOutputs=4  omode=Inherit via internal rule  otype=sfix(16)  scale=2^-15  rndmethod=Unbiased  factor=1  satmethod=Symmetric  shift_vec=[0 1 2 -1]  value=[-26 20 12]  inPortNames=['x';'n']  outPortNames=['r ';'xO';'xU';'aO';]  dspbaimage=dspba_prim_float.jpg  text=fprintf('acc(x)');  style=Optimised  visibilities=1024  version=20090407
  And : DSPBAPrim/And  primtype=and  nInputs=3  nOutputs=1  omode=Inherit via internal rule  otype=sfix(16)  scale=2^-15  rndmethod=Unbiased  factor=1  satmethod=Symmetric  shift_vec=[0 1 2 -1]  value=0  inPortNames=[' '; ' '; ' '; ' '; ' '; ' '; ' '; ' '; ' '; ' '; ' '; ' '; ' '; ' '; ' '; ' '; ]  outPortNames=[' ']  dspbaimage=dspba_prim.jpg  text=fprintf('&');  style=Optimised  visibilities=8+2  version=20090407
  ChannelIn : DSPBAPrim/ChannelIn  primtype=channelin  nInputs=dspba_internal_get_channel_ports(gcb)  nOutputs=dspba_internal_get_channel_ports(gcb)  omode=Inherit via internal rule  otype=sfix(16)  scale=2^-15  rndmethod=Unbiased  factor=1  satmethod=Symmetric  shift_vec=[0 1 2 -1]  value=6  inPortNames=['v'; 'c'; '0'; '1'; '2'; '3'; '4'; '5'; '6'; '7'; '8'; '9'; 'A'; 'B'; 'D'; 'E'; 'F'; 'G'; 'H'; 'I'; 'J'; 'K'; 'L'; 'M'; 'N'; 'O'; 'P'; 'Q'; 'R'; 'S'; 'T'; 'U'; 'W'; 'X'; 'Y'; 'Z']  outPortNames=['v'; 'c'; '0'; '1'; '2'; '3'; '4'; '5'; '6'; '7'; '8'; '9'; 'A'; 'B'; 'D'; 'E'; 'F'; 'G'; 'H'; 'I'; 'J'; 'K'; 'L'; 'M'; 'N'; 'O'; 'P'; 'Q'; 'R'; 'S'; 'T'; 'U'; 'W'; 'X'; 'Y'; 'Z']  dspbaimage=dspba_prim.jpg  text=fprintf('In');  style=Optimised  dataSignals=6  foldingEnabled=off  channels=1  sampleRate=200  packetBeginPresent=off  packetBeginEnabled=off  visibilities=dspba_ChannelInVis(gcb)  latencyCorrection=0  version=20141013
  Complex to Real-Imag : ComplexToRealImag
  Const7 : DSPBAPrim/Const  primtype=const  nInputs=0  nOutputs=1  omode=Specify via dialog  otype=uint(8)  scale=1  rndmethod=Unbiased  factor=1  satmethod=Symmetric  shift_vec=[0 1 2 -1]  value=0  inPortNames=['+'; '+';]  outPortNames=[' ']  dspbaimage=dspba_prim.jpg  text=fprintf('%s', num2str(value));  style=Optimised  visibilities=8 + 1024  floatPrecision=float32_m23  version=20120820
  Demux : Demux  Outputs=2
  Dot Product ChannelOut : DSPBAPrim/ChannelOut  primtype=channelout  nInputs=dspba_internal_get_channel_ports(gcb)  nOutputs=dspba_internal_get_channel_ports(gcb)  omode=Inherit via internal rule  otype=sfix(16)  scale=2^-15  rndmethod=Unbiased  factor=1  satmethod=Symmetric  shift_vec=[0 1 2 -1]  value=1  inPortNames=['v'; 'c'; '0'; '1'; '2'; '3'; '4'; '5'; '6'; '7'; '8'; '9'; 'A'; 'B'; 'D'; 'E'; 'F'; 'G'; 'H'; 'I'; 'J'; 'K'; 'L'; 'M'; 'N'; 'O'; 'P'; 'Q'; 'R'; 'S'; 'T'; 'U'; 'W'; 'X'; 'Y'; 'Z']  outPortNames=['v'; 'c'; '0'; '1'; '2'; '3'; '4'; '5'; '6'; '7'; '8'; '9'; 'A'; 'B'; 'D'; 'E'; 'F'; 'G'; 'H'; 'I'; 'J'; 'K'; 'L'; 'M'; 'N'; 'O'; 'P'; 'Q'; 'R'; 'S'; 'T'; 'U'; 'W'; 'X'; 'Y'; 'Z']  dspbaimage=dspba_prim.jpg  text=fprintf('Out%s', AdvDSPBChannelOutDisplay(latency));  style=Optimised  dataSignals=1  foldingEnabled=off  channels=1  sampleRate=200  packetBeginPresent=off  packetBeginEnabled=off  visibilities=dspba_ChannelOutVis(gcb)  latency=0  latencyCorrection=0  version=20141013
  Mult : DSPBAPrim/Mult  primtype=mult  nInputs=2  nOutputs=1  omode=Inherit via internal rule  otype=sfix(16)  scale=2^-15  rndmethod=Unbiased  factor=1  satmethod=Symmetric  shift_vec=[0 1 2 -1]  value=0  inPortNames=[' '; ' ';]  outPortNames=[' ']  dspbaimage=dspba_prim.jpg  text=fprintf('X');  style=Optimised  visibilities=8+2^18+2^19  floatPrecision=float32_m23  floatRounding=correct  advOptions=[]  version=20130115
  Mult ChannelOut : DSPBAPrim/ChannelOut  primtype=channelout  nInputs=dspba_internal_get_channel_ports(gcb)  nOutputs=dspba_internal_get_channel_ports(gcb)  omode=Inherit via internal rule  otype=sfix(16)  scale=2^-15  rndmethod=Unbiased  factor=1  satmethod=Symmetric  shift_vec=[0 1 2 -1]  value=1  inPortNames=['v'; 'c'; '0'; '1'; '2'; '3'; '4'; '5'; '6'; '7'; '8'; '9'; 'A'; 'B'; 'D'; 'E'; 'F'; 'G'; 'H'; 'I'; 'J'; 'K'; 'L'; 'M'; 'N'; 'O'; 'P'; 'Q'; 'R'; 'S'; 'T'; 'U'; 'W'; 'X'; 'Y'; 'Z']  outPortNames=['v'; 'c'; '0'; '1'; '2'; '3'; '4'; '5'; '6'; '7'; '8'; '9'; 'A'; 'B'; 'D'; 'E'; 'F'; 'G'; 'H'; 'I'; 'J'; 'K'; 'L'; 'M'; 'N'; 'O'; 'P'; 'Q'; 'R'; 'S'; 'T'; 'U'; 'W'; 'X'; 'Y'; 'Z']  dspbaimage=dspba_prim.jpg  text=fprintf('Out%s', AdvDSPBChannelOutDisplay(latency));  style=Optimised  dataSignals=1  foldingEnabled=off  channels=1  sampleRate=200  packetBeginPresent=off  packetBeginEnabled=off  visibilities=dspba_ChannelOutVis(gcb)  latency=0  latencyCorrection=0  version=20141013
  Mux : Mux  Inputs=2
  Real-Imag to Complex : RealImagToComplex
  ReinterpretCast : DSPBAPrim/ReinterpretCast  primtype=reinterpret  nInputs=1  nOutputs=1  omode=single  otype=sfix(16)  scale=2^-15  rndmethod=Unbiased  factor=1  satmethod=Symmetric  shift_vec=[0 1 2 -1]  value=0  inPortNames=[' '; ' ';]  outPortNames=[' ']  dspbaimage=dspba_prim.jpg  text=fprintf('Reinterp\nCast', value);  style=Optimised  visibilities=8  floatPrecision=float32_m23  version=20120601
  ReinterpretCast1 : DSPBAPrim/ReinterpretCast  primtype=reinterpret  nInputs=1  nOutputs=1  omode=single  otype=sfix(16)  scale=2^-15  rndmethod=Unbiased  factor=1  satmethod=Symmetric  shift_vec=[0 1 2 -1]  value=0  inPortNames=[' '; ' ';]  outPortNames=[' ']  dspbaimage=dspba_prim.jpg  text=fprintf('Reinterp\nCast', value);  style=Optimised  visibilities=8  floatPrecision=float32_m23  version=20120601
  SynthesisInfo : DSPBAPrim/SynthesisInfo  primtype=synthinfo  nInputs=0  nOutputs=0  omode=Inherit via internal rule  otype=sfix(16)  scale=2^-15  rndmethod=Truncate  factor=1  satmethod=Symmetric  shift_vec=[0 1 2 -1]  value=99  inPortNames=[' '; ' ';]  outPortNames=[' ']  dspbaimage=dspba_prim_ctrl.jpg  text=fprintf('Style=%s', style);  style=Scheduled  visibilities=2^17+2^18+2^19+2^20  constraintInUse=off  constraintRelation=>  constraintLimit=2  bitAccurate=off  version=20150220
  latch_0L : DSPBAControl/latch_0L
  Dot Product Valid_Out : Outport
  Dot Product Data_Out : Outport  Port=2
  Mult Valid_out : Outport  Port=3
  Mult Data_out : Outport  Port=4
  wires:
  latch_0L/1 -> Dot Product ChannelOut/3
  ReinterpretCast/1 -> latch_0L/2
  ChannelIn/8 -> Mult ChannelOut/1
  Mult ChannelOut/3 -> Mult Data_out/1
  Mult ChannelOut/1 -> Mult Valid_out/1
  ChannelIn/1 -> And/1
  Const7/1 -> Mult ChannelOut/2
  ChannelIn/2 -> Dot Product ChannelOut/2
  Data_In2/1 -> ChannelIn/4
  Dot Product ChannelOut/3 -> Dot Product Data_Out/1
  Dot Product ChannelOut/1 -> Dot Product Valid_Out/1
  ChannelIn/3 -> Mult/1
  Demux/1 -> Real-Imag to Complex/1
  Acc_Valid/1 -> ChannelIn/6
  Complex to Real-Imag/1 -> Mux/1
  Acc_Init/1 -> ChannelIn/5
  Real-Imag to Complex/1 -> ReinterpretCast/1
  Mult/1 -> Complex to Real-Imag/1, ReinterpretCast1/1
  Complex to Real-Imag/2 -> Mux/2
  Channel_In/1 -> ChannelIn/2
  ChannelIn/4 -> Mult/2
  Acc/1 -> Demux/1
  Mux/1 -> Acc/1
  Demux/2 -> Real-Imag to Complex/2
  ChannelIn/5 -> Acc/2
  Valid_In/1 -> ChannelIn/1
  Data_In1/1 -> ChannelIn/3
  ChannelIn/6 -> And/2, latch_0L/1
  And/1 -> Dot Product ChannelOut/1
  Mult_Valid_In/1 -> ChannelIn/8
  ReinterpretCast1/1 -> Mult ChannelOut/3
  Dot_Product_Valid_In/1 -> ChannelIn/7
  ChannelIn/7 -> And/3

== system qrd_matrix_library/Back_Substitution/Input Memory Controller ==
  Z External Write : Inport
  Z External Write Address : Inport  Port=2
  Z External Write Data : Inport  Port=3
  Z Read Address : Inport  Port=4
  Inv Rk External Write : Inport  Port=5
  Inv Rk External Write Address : Inport  Port=6
  Inv Rk External Write Data : Inport  Port=7
  Inv Rk Read Address : Inport  Port=8
  Rn External Write : Inport  Port=9
  Rn External Write Address : Inport  Port=10
  Rn External Write Data : Inport  Port=11
  Rn Read Address : Inport  Port=12
  Inv Rk Input RAM : DSPBAPrim/DualMem  primtype=dualmem  nInputs=4  nOutputs=2  omode=Inherit via internal rule  otype=sfix(16)  scale=2^-15  rndmethod=Unbiased  factor=1  satmethod=Symmetric  shift_vec=[0 1 2 -1]  value=(zeros(size,1))  inPortNames=['d1'; 'a1'; 'w1'; 'a2']  outPortNames=['q1'; 'q2']  dspbaimage=dspba_prim.jpg  text=fprintf('dmem%s',AdvDSPBDMemDisplay(UseDontCare));  style=Optimised  visibilities=8 + 1024 + 2^17 + 2^18  UseDontCare=on  TwinWritePorts=off  version=20141001
  Rn Input RAM : DSPBAPrim/DualMem  primtype=dualmem  nInputs=4  nOutputs=2  omode=Inherit via internal rule  otype=sfix(16)  scale=2^-15  rndmethod=Unbiased  factor=1  satmethod=Symmetric  shift_vec=[0 1 2 -1]  value=complex(zeros(((size-1)*size/2),1),zeros(((size-1)*size/2),1))  inPortNames=['d1'; 'a1'; 'w1'; 'a2']  outPortNames=['q1'; 'q2']  dspbaimage=dspba_prim.jpg  text=fprintf('dmem%s',AdvDSPBDMemDisplay(UseDontCare));  style=Optimised  visibilities=8 + 1024 + 2^17 + 2^18  UseDontCare=on  TwinWritePorts=off  version=20141001
  Z Input RAM : DSPBAPrim/DualMem  primtype=dualmem  nInputs=4  nOutputs=2  omode=Inherit via internal rule  otype=sfix(16)  scale=2^-15  rndmethod=Unbiased  factor=1  satmethod=Symmetric  shift_vec=[0 1 2 -1]  value=complex(zeros(size,instances),zeros(size,instances))  inPortNames=['d1'; 'a1'; 'w1'; 'a2']  outPortNames=['q1'; 'q2']  dspbaimage=dspba_prim.jpg  text=fprintf('dmem%s',AdvDSPBDMemDisplay(UseDontCare));  style=Optimised  visibilities=8 + 1024 + 2^17 + 2^18  UseDontCare=on  TwinWritePorts=off  version=20141001
  Z Data : Outport
  Inv Rk Data : Outport  Port=2
  Rn Data : Outport  Port=3
  wires:
  Z Read Address/1 -> Z Input RAM/4
  Z External Write Address/1 -> Z Input RAM/2
  Z External Write Data/1 -> Z Input RAM/1
  Z External Write/1 -> Z Input RAM/3
  Inv Rk Read Address/1 -> Inv Rk Input RAM/4
  Z Input RAM/2 -> Z Data/1
  Inv Rk Input RAM/2 -> Inv Rk Data/1
  Inv Rk External Write/1 -> Inv Rk Input RAM/3
  Inv Rk External Write Address/1 -> Inv Rk Input RAM/2
  Inv Rk External Write Data/1 -> Inv Rk Input RAM/1
  Rn Read Address/1 -> Rn Input RAM/4
  Rn Input RAM/2 -> Rn Data/1
  Rn External Write/1 -> Rn Input RAM/3
  Rn External Write Address/1 -> Rn Input RAM/2
  Rn External Write Data/1 -> Rn Input RAM/1

== system qrd_matrix_library/Back_Substitution/Output Memory Controller ==
  Write Enable : Inport
  Write Address : Inport  Port=2
  Write Data : Inport  Port=3
  Read Valid 1 : Inport  Port=4
  Read Address 1 : Inport  Port=5
  Read Valid 2 : Inport  Port=6
  Read Address 2 : Inport  Port=7
  Const : DSPBAPrim/Const  primtype=const  nInputs=0  nOutputs=1  omode=Inherit via internal rule  otype=sfix(16)  scale=2^-15  rndmethod=Unbiased  factor=1  satmethod=Symmetric  shift_vec=[0 1 2 -1]  value=0  inPortNames=['+'; '+';]  outPortNames=[' ']  dspbaimage=dspba_prim.jpg  text=fprintf('%s', num2str(value));  style=Optimised  visibilities=8 + 1024  floatPrecision=float32_m23  version=20120820
  Result RAM : DSPBAPrim/DualMem  primtype=dualmem  nInputs=4  nOutputs=2  omode=Inherit via internal rule  otype=sfix(16)  scale=2^-15  rndmethod=Unbiased  factor=1  satmethod=Symmetric  shift_vec=[0 1 2 -1]  value=complex(zeros(size,instances),zeros(size,instances))  inPortNames=['d1'; 'a1'; 'w1'; 'a2']  outPortNames=['q1'; 'q2']  dspbaimage=dspba_prim.jpg  text=fprintf('dmem%s',AdvDSPBDMemDisplay(UseDontCare));  style=Optimised  visibilities=8 + 1024 + 2^17 + 2^18  UseDontCare=on  TwinWritePorts=off  version=20141001
  Select : DSPBAPrim/Select  primtype=select  nInputs=str2num(get_param(gcb,'value'))*2+1  nOutputs=1  omode=Inherit via internal rule  otype=sfix(16)  scale=2^-15  rndmethod=Unbiased  factor=1  satmethod=Symmetric  shift_vec=[0 1 2 -1]  value=2  inPortNames=['d'; '0'; 'a'; '1'; 'b'; '2'; 'c'; '3'; 'd'; '4'; 'e'; '5'; 'f'; '6'; 'g'; '7'; 'h'; '8'; 'i'; '9'; 'j']  outPortNames=[' ']  dspbaimage=dspba_prim.jpg  text=fprintf('%s', primtype);  style=Optimised  visibilities=8 + 1024  version=20090407
  Read Data : Outport
  wires:
  Write Address/1 -> Result RAM/2
  Write Data/1 -> Result RAM/1
  Read Address 1/1 -> Select/3
  Result RAM/2 -> Read Data/1
  Write Enable/1 -> Result RAM/3
  Read Address 2/1 -> Select/5
  Select/1 -> Result RAM/4
  Read Valid 1/1 -> Select/2
  Read Valid 2/1 -> Select/4
  Const/1 -> Select/1
